simulink model "SMDFR_HTE_model"  (R2024b)
settings: Solver=ode15s  StartTime=1  StopTime=1200  FixedStep=0.01  RelTol=1e-3
model workspace (MAT data in the model file):
  ACS_lambda = 0.000161129786201
  A_cucl = 134.446
  A_cucl2 = 134.446
  A_cuocl = 213.991
  A_d = 217.647058824
  A_fw = [13.6 90 13.6]
  A_h = 217.647058824
  A_h2 = 217.647058824
  A_h20 = 18.015
  A_hcl = 36.458
  A_o = 32
  A_sg = 370
  A_wc = [10.9 103 10.9]
  C_c = 140.2
  C_cucl = 0.71
  C_cuocl = 1
  C_dst = 1996000
  C_h20 = 4.48
  C_hcl = 0.8
  C_hst = 1996000
  C_i0 = [429000000000000; 4.15e+15; 3.83e+15; 1.16e+16; 5.7e+15; 1.53e+15]
  C_o = 0.918
  Ce_i0 = [701000000000000; 5.88e+15; 3.36e+15; 5.09e+15; 820000000000000; 39600000000000]
  Cr = 0.00113148387097
  Cr_m = 8.769
  Cr_m_red = 4.3845
  Cr_red = 0.000565741935484
  D = 0.16
  DPB_lambda = 0.01
  EPB_lambda = 0.01
  E_d = 5
  E_e = 5
  E_h = 5
  E_hte = 5
  G_cucl = 44.778
  G_cucl2 = 44.778
  G_cuocl = 35.6355
  G_h2 = 32
  G_h20 = 10
  G_h20i = 10
  G_h20o = 7
  G_hcl = 12.1426
  G_o = 2.66
  G_s = 27000
  H_valve = 1
  Heat = [18744000 5970000 16956000]
  IPB_lambda = 0.01
  K_d = 500
  K_h = 500
  L = 6
  LOCA1 = 0
  LOCA2 = 0
  LOCA3 = 0
  LOCA4 = 0
  LOCA_p = 0.000161129786201
  LOCA_time = 300
  LOCA_times = [408 453 64 457 317 49 140 274 479 483 79 486 ... (4000 elements, 1000x4)]
  LOPC = 0
  LOPC_p = 0.1
  LOPC_times = [214 478 363 291 271 353 3 392 464 5 413 384 ... (1000 elements, 1000x1)]
  L_ACS = 0.01
  Lambda = 1.05e-06
  M_c = [219.9 7705 219.9]
  M_cucl0 = 44.778
  M_cucl20 = 44.778
  M_f = [307.7 1164 307.7]
  M_h20 = 8
  M_hcl0 = 12.1426
  M_w = [39.3 311 39.3]
  N = 1000
  N_0 = 15000000000000
  Nodes = 3
  P_0 = 100000000
  P_decomposition = 160
  P_hydro = 167
  Pb_acs : object (value not decoded)
  Pb_pipes : object (value not decoded)
  Pi_0 = [0.158 0.6899 0.152]
  Power_lambda = 0.01
  RPB_lambda = 0.01
  T_fw = 300
  T_hpi = 100
  T_st = 900
  Tbar_c0 = 1060
  Tbar_f0 = 1288
  Tc_in = 973
  Tin_c = 973
  Tin_f = 1300
  Tout_c = 1100
  Tout_f = 1300
  V_c = 160
  V_d = 160
  V_dst = 100
  V_h = 160
  V_h2 = 160
  V_hst = 100
  V_s = 100
  V_sg = 100
  age = 0
  ages = [0 50]
  alfa_c = -8.28e-06
  alfa_f = -0.000208
  alpha = 0.9926
  alpha_1 = 1
  alpha_2 = 1
  alpha_3 = 1
  alpha_4 = 1
  beta = 0.00302
  beta_i = [7.91e-05 0.000703 0.000504 0.00117 0.000457 0.00011]
  c_pc = [140.2 140.2 140.2]
  c_pf = [400 400 400]
  c_pw = [690 690 690]
  coolpipes = [2166 2166 0]
  d_c = 10187.40024
  d_dst = 3.14
  d_hst = 3.14
  d_st = 6.123
  demand = [0.661834040547 0.662423385196 0.661244695898 0.663602074493 0.660066006601 0.661244695898 0.662423385196 0.662423385196 0.662423385196 0.661244695898 0.661244695898 0.661244695898 ... (8761 elements, 8761x1)]
  diesel_lambda = 0.01
  eta = 0.4
  fail_threshold = 1244
  file = 'SMDFR_Parameters'
  fuelpipes = 1027
  h_dpo = 6801000
  h_fw = [6546 4305.1 7629.5]
  h_fw_st = 4386450
  h_hpo = 7159680
  h_in = 7000
  h_out = 1000
  h_st_in = 4386450
  h_wc = [27405.4 13833.4 32177.3]
  i = 1
  j = 1
  k_d = 2.7187
  k_e = 2.7187
  k_h = 0.005
  k_hte = 2.7187
  k_sg = 500
  lambda_c = 0.184
  lambda_e = 0.1
  lambda_i = [0.0127 0.03 0.11 0.319 1.18 7.02]
  leakage = 6.5
  mdot_c = [5550.5 5550.5 5550.5]
  mdot_c_value = 5550.5
  mdot_f = [327.7 327.7 327.7]
  mdot_f_value = 327.7
  model = 'SMDFR'
  mu = 50.9722799688
  mu_f = -20.9722799688
  mu_o = 30
  n = 0.45
  nsim = 1
  p_h20 = 40
  phi_tot = 3.61e+21
  rho = 7750
  rho_0 = 0.00111
  rhoex_value = 0
  sigma = 625
  sigma_c = 5
  sigma_f = 5.83095189485
  sigma_o = 3
  step = 0.1
  t = 0.008
  tau_c = 5.43
  tau_e = 10
  tr_fun = cfit
  tr_fun.coeffValues{1}.form = 'pp'
  tr_fun.coeffValues{1}.breaks = [0 34473.8 55158.08 82737.12 122381.99]
  tr_fun.coeffValues{1}.coefs = [2.32060289263e-05  0; 5.70481544439e-06  0.8; 2.97327245618e-06  0.918; 0  1]
  tr_fun.coeffValues{1}.pieces = 4
  tr_fun.coeffValues{1}.order = 2
  tr_fun.coeffValues{1}.dim = 1
  tr_fun.sse = 0
  tr_fun.dfe = 0
  tr_fun.activebounds = 0
  tr_fun.xlim = [0 122381.99]
  tr_fun.fittype.fType = 'linearinterp'
  tr_fun.fittype.fTypename = 'Linear interpolant'
  tr_fun.fittype.fCategory = 'interpolant'
  tr_fun.fittype.defn = 'piecewise polynomial'
  tr_fun.fittype.fFeval = 1
  tr_fun.fittype.args = ['p'; 'x']
  tr_fun.fittype.isEmpty = 0
  tr_fun.fittype.numArgs = 2
  tr_fun.fittype.indep = 'x'
  tr_fun.fittype.depen = 'y'
  tr_fun.fittype.coeff = 'p'
  tr_fun.fittype.fFitoptions = curvefit.linearinterpoptions
  tr_fun.fittype.fFitoptions.ExtrapolationMethod = 'linear'
  tr_fun.fittype.fFitoptions.Method = 'LinearInterpolant'
  tsim = 500
  turbine_fun = cfit
  turbine_fun.coeffValues{1}.form = 'pp'
  turbine_fun.coeffValues{1}.breaks = [0 4067.9084 6687.9172 10273.1924 14892.6816]
  turbine_fun.coeffValues{1}.coefs = [0  0; 1.52671242936e-07  0; 1.17145819099e-06  0.0004; 7.66318492529e-06  0.0046]
  turbine_fun.coeffValues{1}.pieces = 4
  turbine_fun.coeffValues{1}.order = 2
  turbine_fun.coeffValues{1}.dim = 1
  turbine_fun.sse = 0
  turbine_fun.dfe = 0
  turbine_fun.activebounds = 0
  turbine_fun.xlim = [0 14892.6816]
  turbine_fun.fittype.fType = 'linearinterp'
  turbine_fun.fittype.fTypename = 'Linear interpolant'
  turbine_fun.fittype.fCategory = 'interpolant'
  turbine_fun.fittype.defn = 'piecewise polynomial'
  turbine_fun.fittype.fFeval = 1
  turbine_fun.fittype.args = ['p'; 'x']
  turbine_fun.fittype.isEmpty = 0
  turbine_fun.fittype.numArgs = 2
  turbine_fun.fittype.indep = 'x'
  turbine_fun.fittype.depen = 'y'
  turbine_fun.fittype.coeff = 'p'
  turbine_fun.fittype.fFitoptions = curvefit.linearinterpoptions
  turbine_fun.fittype.fFitoptions.ExtrapolationMethod = 'linear'
  turbine_fun.fittype.fFitoptions.Method = 'LinearInterpolant'
  v_rec = 4.16e-09
values from neighbouring files (symbols this model uses):
  ACS1_flow = 25    [Only_Inputs.m]    (also in Simulation_model.m; Simulation_model_complete.m; Simulation_model_hydrogen.m; Simulation_model_hydrogen_parallel.m)
  ACS1_response_time = randi(t_max_r_ACS-t_min_r_ACS)+t_min_r_ACS    [Failure_model.m]    (also in Failure_model_outputs.mat = 36; Only_Inputs.m = ACS1_response_time(indexes))
  ACS2_flow = 25    [Only_Inputs.m]    (also in Simulation_model.m; Simulation_model_complete.m; Simulation_model_hydrogen.m; Simulation_model_hydrogen_parallel.m)
  ACS2_response_time = randi(t_max_r_ACS-t_min_r_ACS)+t_min_r_ACS    [Failure_model.m]    (also in Failure_model_outputs.mat = 49; Only_Inputs.m = ACS2_response_time(indexes); Simulation_model_hydrogen_parallel.m = 0)
  ACS3_flow = 25    [Only_Inputs.m]    (also in Simulation_model.m; Simulation_model_complete.m; Simulation_model_hydrogen.m; Simulation_model_hydrogen_parallel.m)
  ACS3_response_time = randi(t_max_r_ACS-t_min_r_ACS)+t_min_r_ACS    [Failure_model.m]    (also in Failure_model_outputs.mat = 62; Only_Inputs.m = ACS3_response_time(indexes); Simulation_model_hydrogen_parallel.m = 0)
  ACS4_flow = 25    [Only_Inputs.m]    (also in Simulation_model.m; Simulation_model_complete.m; Simulation_model_hydrogen.m; Simulation_model_hydrogen_parallel.m)
  ACS4_response_time = randi(t_max_r_ACS-t_min_r_ACS)+t_min_r_ACS    [Failure_model.m]    (also in Failure_model_outputs.mat = 57; Only_Inputs.m = ACS4_response_time(indexes); Simulation_model_hydrogen_parallel.m = 0)
  ACS_1 = 821    [Failure_model_outputs.mat]    (also in Failure_sim.m = ACS_times(1); Only_Inputs.m = ACS_1(indexes))
  ACS_2 = 1010    [Failure_model_outputs.mat]    (also in Failure_sim.m = ACS_times(2); Only_Inputs.m = ACS_2(indexes); Simulation_model_hydrogen_parallel.m = 1)
  ACS_3 = 926    [Failure_model_outputs.mat]    (also in Failure_sim.m = ACS_times(3); Only_Inputs.m = ACS_3(indexes); Simulation_model_hydrogen_parallel.m = 1)
  ACS_4 = 80    [Failure_model_outputs.mat]    (also in Failure_sim.m = ACS_times(4); Only_Inputs.m = ACS_4(indexes); Simulation_model_hydrogen_parallel.m = 1)
  All_Outputs = 1    [Only_Inputs.m]    (also in Simulation_model.m = 0; Simulation_model_complete.m = 0; Simulation_model_hydrogen.m = 0; Simulation_model_hydrogen_parallel.m = 0)
  EDG1_response_time = randi(t_max_r_EDG-t_min_r_EDG)+t_min_r_EDG    [Failure_model.m]    (also in Failure_model_outputs.mat = 170; Only_Inputs.m = EDG1_response_time(indexes))
  EDG2_response_time = randi(t_max_r_EDG-t_min_r_EDG)+t_min_r_EDG    [Failure_model.m]    (also in Failure_model_outputs.mat = 133; Only_Inputs.m = EDG2_response_time(indexes); Simulation_model_hydrogen_parallel.m = 0)
  EDG_1 = 567    [Failure_model_outputs.mat]    (also in Only_Inputs.m = EDG_1(indexes))
  EDG_2 = 323    [Failure_model_outputs.mat]    (also in Only_Inputs.m = EDG_2(indexes); Simulation_model_hydrogen_parallel.m = 1)
  LHS = 0    [Failure_model_outputs.mat]    (also in Failure_sim.m = 60; Only_Inputs.m = LHS(indexes))
  LOCA1_time = 1200    [Failure_model_outputs.mat]    (also in Failure_sim.m = loca_times(1); Only_Inputs.m = LOCA1_time(indexes))
  LOCA2_time = 1200    [Failure_model_outputs.mat]    (also in Failure_sim.m = loca_times(2); Only_Inputs.m = LOCA2_time(indexes); Simulation_model_hydrogen_parallel.m)
  LOCA3_time = 39    [Failure_model_outputs.mat]    (also in Failure_sim.m = loca_times(3); Only_Inputs.m = LOCA3_time(indexes); Simulation_model_hydrogen_parallel.m = 1200)
  LOCA4_time = 18    [Failure_model_outputs.mat]    (also in Failure_sim.m = loca_times(4); Only_Inputs.m = LOCA4_time(indexes); Simulation_model_hydrogen_parallel.m = 1200)
  MSLB1 = 1200    [Failure_model_outputs.mat]    (also in Failure_sim.m = fix(randsample(x_loca, 1, true, lognorm_pdf)); Only_Inputs.m = MSLB1(indexes))
  MSLB2 = 1200    [Failure_model_outputs.mat]    (also in Failure_sim.m = fix(randsample(x_loca, 1, true, lognorm_pdf)); Only_Inputs.m = MSLB2(indexes); Simulation_model_hydrogen_parallel.m = 0)
  MSLB3 = 1200    [Failure_model_outputs.mat]    (also in Failure_sim.m = fix(randsample(x_loca, 1, true, lognorm_pdf)); Only_Inputs.m = MSLB3(indexes); Simulation_model_hydrogen_parallel.m = 0)
  MSLB4 = 1200    [Failure_model_outputs.mat]    (also in Failure_sim.m = fix(randsample(x_loca, 1, true, lognorm_pdf)); Only_Inputs.m = MSLB4(indexes); Simulation_model_hydrogen_parallel.m = 0)
  PDP11 = 1200    [Failure_model_outputs.mat]    (also in Failure_sim.m = pdp_times(1); Only_Inputs.m = PDP11(indexes))
  PDP11_response_time = randi(t_max_r_EDG-t_min_r_EDG)+t_min_r_EDG    [Failure_model.m]    (also in Failure_model_outputs.mat = 136; Only_Inputs.m = PDP11_response_time(indexes))
  PDP12 = 1200    [Failure_model_outputs.mat]    (also in Failure_sim.m = pdp_times(2); Only_Inputs.m = PDP12(indexes); Simulation_model_hydrogen_parallel.m = 0)
  PDP12_response_time = randi(t_max_r_EDG-t_min_r_EDG)+t_min_r_EDG    [Failure_model.m]    (also in Failure_model_outputs.mat = 119; Only_Inputs.m = PDP12_response_time(indexes); Simulation_model_hydrogen_parallel.m = 0)
  PDP21 = 1200    [Failure_model_outputs.mat]    (also in Failure_sim.m = pdp_times(3); Only_Inputs.m = PDP21(indexes); Simulation_model_hydrogen_parallel.m = 0)
  PDP21_response_time = randi(t_max_r_EDG-t_min_r_EDG)+t_min_r_EDG    [Failure_model.m]    (also in Failure_model_outputs.mat = 17; Only_Inputs.m = PDP21_response_time(indexes); Simulation_model_hydrogen_parallel.m = 0)
  PDP22 = 1200    [Failure_model_outputs.mat]    (also in Failure_sim.m = pdp_times(4); Only_Inputs.m = PDP22(indexes); Simulation_model_hydrogen_parallel.m = 0)
  PDP22_response_time = randi(t_max_r_EDG-t_min_r_EDG)+t_min_r_EDG    [Failure_model.m]    (also in Failure_model_outputs.mat = 120; Only_Inputs.m = PDP22_response_time(indexes); Simulation_model_hydrogen_parallel.m = 0)
  PDP31 = 1200    [Failure_model_outputs.mat]    (also in Failure_sim.m = pdp_times(5); Only_Inputs.m = PDP31(indexes); Simulation_model_hydrogen_parallel.m = 0)
  PDP31_response_time = randi(t_max_r_EDG-t_min_r_EDG)+t_min_r_EDG    [Failure_model.m]    (also in Failure_model_outputs.mat = 65; Only_Inputs.m = PDP31_response_time(indexes); Simulation_model_hydrogen_parallel.m = 0)
  PDP32 = 1200    [Failure_model_outputs.mat]    (also in Failure_sim.m = pdp_times(6); Only_Inputs.m = PDP32(indexes); Simulation_model_hydrogen_parallel.m = 0)
  PDP32_response_time = randi(t_max_r_EDG-t_min_r_EDG)+t_min_r_EDG    [Failure_model.m]    (also in Failure_model_outputs.mat = 28; Only_Inputs.m = PDP32_response_time(indexes); Simulation_model_hydrogen_parallel.m = 0)
  PDP41 = 1200    [Failure_model_outputs.mat]    (also in Failure_sim.m = pdp_times(7); Only_Inputs.m = PDP41(indexes); Simulation_model_hydrogen_parallel.m = 0)
  PDP41_response_time = randi(t_max_r_EDG-t_min_r_EDG)+t_min_r_EDG    [Failure_model.m]    (also in Failure_model_outputs.mat = 24; Only_Inputs.m = PDP41_response_time(indexes); Simulation_model_hydrogen_parallel.m = 0)
  PDP42 = 1200    [Failure_model_outputs.mat]    (also in Failure_sim.m = pdp_times(8); Only_Inputs.m = PDP42(indexes); Simulation_model_hydrogen_parallel.m = 0)
  PDP42_response_time = randi(t_max_r_EDG-t_min_r_EDG)+t_min_r_EDG    [Failure_model.m]    (also in Failure_model_outputs.mat = 164; Only_Inputs.m = PDP42_response_time(indexes); Simulation_model_hydrogen_parallel.m = 0)
  PGA = zeros(N,1)    [Crude_MC.m]    (also in Failure_model_outputs.mat = 0.3; Only_Inputs.m = PGA(indexes); Results.mat = [0.197697697698 0.158618618619 0.354014014014 0.1 0.1 0.4126; Simulation_model_hydrogen_parallel.m = 0)
  Power = 1200    [Failure_model_outputs.mat]    (also in Failure_sim.m = fix(randsample(x_loca, 1, true, lognorm_pdf)); Only_Inputs.m = Power(indexes))
  thermal_failure = 0    [Failure_model_outputs.mat]    (also in Failure_sim.m = 1; Only_Inputs.m = zeros(N,1); Simulation_model_hydrogen_parallel.m)
  thermal_failure_time = 1200    [Failure_model_outputs.mat]    (also in Failure_sim.m = 60; Only_Inputs.m = zeros(N,1); Simulation_model_hydrogen_parallel.m)
libraries: SMDFR_lib x8
(part 1 of 2)
settings Model: Creator=leona  LastModifiedBy=stefanomarchetti
settings OptimizationCC: ReuseModelBlockBuffer=off
settings DebuggingCC: UnconnectedInputMsg=warning  UnconnectedLineMsg=warning
settings ModelReferenceCC: EnableRefExpFcnMdlSchedulingChecks=on
settings RTWCC: GPUComputeCapability=3.5  DLArmComputeVersion=19.05

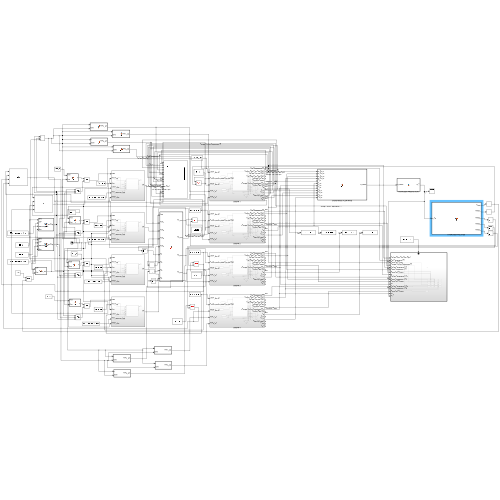
[thumbnail: Simulink's stored preview of the top-level diagram]
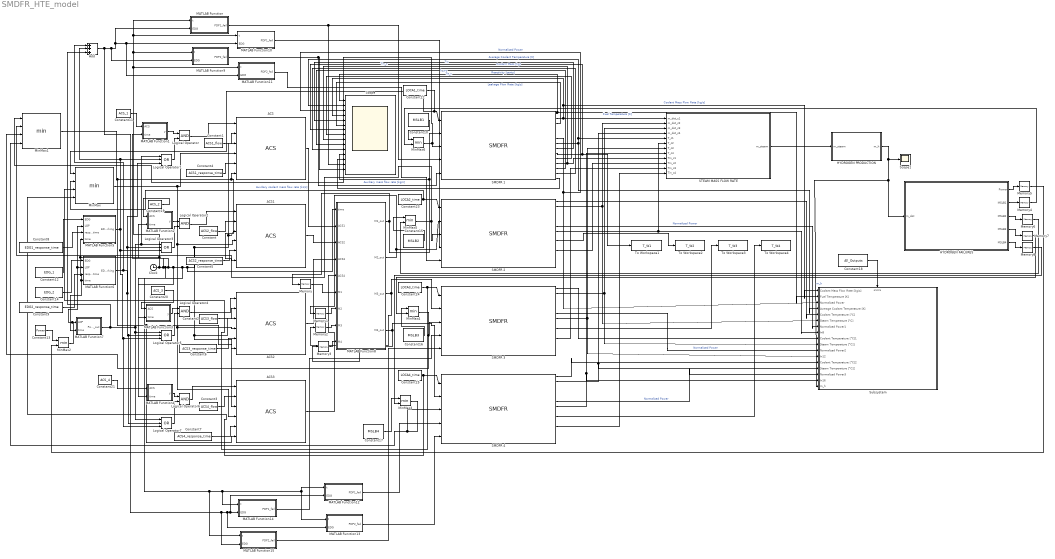
== system SMDFR_HTE_model ==
  ACS{,1..3} (4 alike) : SMDFR_lib/ACS  SystemSampleTime=-1  VariantActivationTime=update diagram  AllowFlexibleInterface=on  Latency=0  AutoFrameSizeCalculation=off
  Add : Sum  Inputs=+++
  Clock : Clock
  Constant : Constant  Value=ACS2_flow
  Constant1 : Constant  Value=ACS1_flow
  Constant10 : Constant  Value=MSLB1
  Constant11 : Constant  Value=ACS_1
  Constant12 : Constant  Value=EDG_1
  Constant13 : Constant  Value=Power
  Constant14 : Constant  Value=EDG_2
  Constant15 : Constant  Value=MSLB2
  Constant16 : Constant  Value=MSLB3
  Constant17 : Constant  Value=MSLB4
  Constant18 : Constant  Value=All_Outputs
  Constant19 : Constant  Value=ACS_2
  Constant2 : Constant  Value=ACS3_flow
  Constant20 : Constant  Value=ACS_3
  Constant21 : Constant  Value=ACS_4
  Constant22 : Constant  Value=LOCA1_time
  Constant23 : Constant  Value=LOCA2_time
  Constant24 : Constant  Value=LOCA3_time
  Constant25 : Constant  Value=LOCA4_time
  Constant3 : Constant  Value=ACS4_flow
  Constant4 : Constant  Value=ACS1_response_time
  Constant5 : Constant  Value=ACS2_response_time
  Constant6 : Constant  Value=ACS3_response_time
  Constant7 : Constant  Value=ACS4_response_time
  Constant8 : Constant  Value=EDG1_response_time
  Constant9 : Constant  Value=EDG2_response_time
  HYDROGEN FAILURES : MATLAB Function  TreatAsAtomicUnit=on
  HYDROGEN PRODUCTION : MATLAB Function  TreatAsAtomicUnit=on
  Logical Operator{,2,4,6} (4 alike) : Logic  AllPortsSameDT=off  OutDataTypeStr=boolean
  Logical Operator{1,3,5,7} (4 alike) : Logic  Operator=OR  Inputs=3  AllPortsSameDT=off  OutDataTypeStr=boolean
  MATLAB Function : MATLAB Function  TreatAsAtomicUnit=on
  MATLAB Function1 : MATLAB Function  TreatAsAtomicUnit=on
  MATLAB Function10 : MATLAB Function  TreatAsAtomicUnit=on
  MATLAB Function11 : MATLAB Function  TreatAsAtomicUnit=on
  MATLAB Function12 : MATLAB Function  TreatAsAtomicUnit=on
  MATLAB Function13 : MATLAB Function  TreatAsAtomicUnit=on
  MATLAB Function14 : MATLAB Function  TreatAsAtomicUnit=on
  MATLAB Function15 : MATLAB Function  TreatAsAtomicUnit=on
  MATLAB Function2 : MATLAB Function  TreatAsAtomicUnit=on
  MATLAB Function3 : MATLAB Function  TreatAsAtomicUnit=on
  MATLAB Function4 : MATLAB Function  TreatAsAtomicUnit=on
  MATLAB Function5 : MATLAB Function  TreatAsAtomicUnit=on
  MATLAB Function6 : MATLAB Function  TreatAsAtomicUnit=on
  MATLAB Function7 : MATLAB Function  TreatAsAtomicUnit=on
  MATLAB Function8 : MATLAB Function  TreatAsAtomicUnit=on
  MATLAB Function9 : MATLAB Function  TreatAsAtomicUnit=on
  Memory{,1..8} (9 alike) : Memory
  MinMax : MinMax  Inputs=4
  MinMax1 : MinMax  Inputs=4
  MinMax{2..6} (5 alike) : MinMax  Inputs=2
  SMDFR 1 : SMDFR_lib/SMDFR  SystemSampleTime=-1  VariantActivationTime=update diagram  AllowFlexibleInterface=on  Latency=0  AutoFrameSizeCalculation=off
  SMDFR 2 : SMDFR_lib/SMDFR  SystemSampleTime=-1  VariantActivationTime=update diagram  AllowFlexibleInterface=on  Latency=0  AutoFrameSizeCalculation=off
      link override SMDFR/SMDFR 1/Constant10: Value=mdot_c_faultcase_2
  SMDFR 3 : SMDFR_lib/SMDFR  SystemSampleTime=-1  VariantActivationTime=update diagram  AllowFlexibleInterface=on  Latency=0  AutoFrameSizeCalculation=off
      link override SMDFR/SMDFR 1/Constant10: Value=mdot_c_faultcase_3
  SMDFR 4 : SMDFR_lib/SMDFR  SystemSampleTime=-1  VariantActivationTime=update diagram  AllowFlexibleInterface=on  Latency=0  AutoFrameSizeCalculation=off
      link override SMDFR/SMDFR 1/Constant10: Value=mdot_c_faultcase_3
  STEAM MASS FLOW RATE : MATLAB Function  TreatAsAtomicUnit=on
  Scope : Scope  NumInputPorts=15
  Scope1 : Scope
  Subsystem : Subsystem
  To Workspace1 : ToWorkspace  VariableName=T_W1  SampleTime=1
  To Workspace2 : ToWorkspace  VariableName=T_W2  SampleTime=1
  To Workspace3 : ToWorkspace  VariableName=T_W3  SampleTime=1
  To Workspace4 : ToWorkspace  VariableName=T_W4  SampleTime=1
  wires:
  SMDFR 1/1 -> Subsystem/2(Fuel Temperature [K]), Scope/1  "Fuel Temperature [K]"
  SMDFR 1/2 -> Subsystem/1(Coolant Mass Flow Rate [kg/s]), Scope/4, STEAM MASS FLOW RATE/1(m_dot_c1)  "Coolant Mass Flow Rate [kg/s]"
  SMDFR 1/6 -> Subsystem/3(Normalized Power), Scope/3  "Normalized Power"
  ACS/1 -> MATLAB Function8/2(ACS1)  "Auxiliary coolant mass flow rate [ks/s]"
  ACS1/1 -> MATLAB Function8/3(ACS2)
  ACS2/1 -> MATLAB Function8/4(ACS3)
  ACS3/1 -> MATLAB Function8/5(ACS4)
  MATLAB Function5/1(EDG_working) -> Logical Operator1/2, Add/2, Logical Operator7/3, Logical Operator5/3, Logical Operator3/3
  Logical Operator1/1 -> Logical Operator/2
  Logical Operator/1 -> ACS/1
  Logical Operator3/1 -> Logical Operator2/2
  MATLAB Function7/1(Power_out) -> Add/3, Logical Operator1/1, Logical Operator3/1, Logical Operator7/1, Logical Operator5/1
  MATLAB Function6/1(EDG_working) -> Add/1, Logical Operator7/2, Logical Operator5/2, Logical Operator1/3, Logical Operator3/2
  Logical Operator2/1 -> ACS1/1
  Logical Operator5/1 -> Logical Operator4/2
  Logical Operator4/1 -> ACS2/1
  Logical Operator7/1 -> Logical Operator6/2
  Logical Operator6/1 -> ACS3/1
  Clock/1 -> MATLAB Function11/1(t), MATLAB Function10/1(t), MATLAB Function/1(t), MATLAB Function9/1(t), MATLAB Function6/4(time), MATLAB Function7/2(time), MATLAB Function5/4(time), MATLAB Function2/2(time), MATLAB Function15/1(t), MATLAB Function14/1(t), MATLAB Function13/1(t), MATLAB Function12/1(t), MATLAB Function1/2(time), MATLAB Function3/2(time), MATLAB Function4/2(time), MATLAB Function8/1(time), ACS1/3, ACS/3, ACS3/3, ACS2/3
  Constant/1 -> ACS1/2
  Constant1/1 -> ACS/2
  Constant2/1 -> ACS2/2
  Constant3/1 -> ACS3/2
  Constant11/1 -> MATLAB Function1/1(ACS)
  Constant19/1 -> MATLAB Function2/1(ACS)
  Constant20/1 -> MATLAB Function3/1(ACS)
  Constant21/1 -> MATLAB Function4/1(ACS)
  Constant22/1 -> MinMax/1, SMDFR 1/1
  Constant23/1 -> SMDFR 2/1, MinMax/2
  Constant24/1 -> MinMax/3, SMDFR 3/1
  Constant25/1 -> SMDFR 4/1, MinMax/4
  MATLAB Function1/1(y) -> Logical Operator/1
  MATLAB Function2/1(y) -> Logical Operator2/1
  MATLAB Function3/1(y) -> Logical Operator4/1
  MATLAB Function4/1(y) -> Logical Operator6/1
  Constant12/1 -> MATLAB Function5/1(EDG)
  Constant14/1 -> MATLAB Function6/1(EDG)
  MinMax2/1 -> MATLAB Function5/2(LOP), MATLAB Function6/2(LOP), MATLAB Function7/1(LOP)
  MATLAB Function8/1(M1_out) -> Memory/1, SMDFR 1/2, Scope/12  "Auxiliary mass flow rate [kg/s]"
  MATLAB Function8/2(M2_out) -> Memory1/1, SMDFR 2/2
  MATLAB Function8/3(M3_out) -> SMDFR 3/2, Memory2/1
  MATLAB Function8/4(M4_out) -> SMDFR 4/2, Memory3/1
  MinMax/1 -> ACS/4, ACS1/4, ACS3/4, ACS2/4
  Constant8/1 -> MATLAB Function5/3(response_time)
  Constant9/1 -> MATLAB Function6/3(response_time)
  Constant4/1 -> ACS/5
  Constant5/1 -> ACS1/5
  Constant6/1 -> ACS2/5
  Constant7/1 -> ACS3/5
  Memory/1 -> MATLAB Function8/6(M1)
  Memory1/1 -> MATLAB Function8/7(M2)
  Memory2/1 -> MATLAB Function8/8(M3)
  Memory3/1 -> MATLAB Function8/9(M4)
  SMDFR 1/7 -> STEAM MASS FLOW RATE/5(T_c1), Scope/2, Subsystem/4(Average Coolant Temperature [K])  "Average Coolant Temperature [K]"
  SMDFR 1/8 -> Scope/5  "Coolant Mass [kg]"
  SMDFR 1/3 -> Scope/6  "Leakage Flow Rate [kg/s]"
  SMDFR 1/9 -> To Workspace1/1, Scope/7  "Tw"
  SMDFR 1/10 -> Scope/8  "Te_c"
  SMDFR 1/11 -> STEAM MASS FLOW RATE/9(Tin_c1), Scope/9  "Tin_c"
  SMDFR 1/12 -> Scope/10  "Reactivity [cents]"
  SMDFR 1/13 -> Scope/11  "h_wc"
  SMDFR 2/9 -> To Workspace2/1
  SMDFR 3/9 -> To Workspace3/1
  SMDFR 4/9 -> To Workspace4/1
  SMDFR 1/14 -> Scope/13
  MATLAB Function/1(PDP1_fail) -> Scope/14, SMDFR 1/4
  MinMax6/1 -> MinMax1/1, SMDFR 1/3
  MinMax5/1 -> SMDFR 2/3, MinMax1/2
  MinMax4/1 -> MinMax1/3, SMDFR 3/3
  MinMax3/1 -> MinMax1/4, SMDFR 4/3
  MATLAB Function10/1(PDP1_fail) -> SMDFR 2/4
  MATLAB Function12/1(PDP1_fail) -> SMDFR 4/4
  MATLAB Function14/1(PDP1_fail) -> SMDFR 3/4
  Add/1 -> MATLAB Function15/2(EDG), MATLAB Function13/2(EDG), MATLAB Function12/2(EDG), MATLAB Function14/2(EDG), MATLAB Function9/2(EDG), MATLAB Function11/2(EDG), MATLAB Function10/2(EDG), MATLAB Function/2(EDG)
  MinMax1/1 -> ACS1/6, ACS/6, ACS2/6, ACS3/6
  MATLAB Function13/1(PDP2_fail) -> SMDFR 4/5
  MATLAB Function15/1(PDP2_fail) -> SMDFR 3/5
  MATLAB Function9/1(PDP2_fail) -> Scope/15, SMDFR 1/5
  MATLAB Function11/1(PDP2_fail) -> SMDFR 2/5
  SMDFR 2/1 -> Subsystem/5(Coolant Temperature [°C])
  SMDFR 2/2 -> STEAM MASS FLOW RATE/2(m_dot_c2), Subsystem/6(Steam Temperature [°C])
  SMDFR 2/6 -> Subsystem/7(Normalized Power1)  "Normalized Power"
  SMDFR 2/7 -> Subsystem/8(In8), STEAM MASS FLOW RATE/6(T_c2)
  SMDFR 3/1 -> Subsystem/9(Coolant Temperature [°C]1)
  SMDFR 3/2 -> STEAM MASS FLOW RATE/3(m_dot_c3), Subsystem/10(Steam Temperature [°C]1)
  SMDFR 3/6 -> Subsystem/11(Normalized Power2)  "Normalized Power"
  SMDFR 3/7 -> STEAM MASS FLOW RATE/7(T_c3), Subsystem/12(In12)
  SMDFR 4/1 -> Subsystem/13(Coolant Temperature [°C]2)
  SMDFR 4/2 -> STEAM MASS FLOW RATE/4(m_dot_c4), Subsystem/14(Steam Temperature [°C]2)
  SMDFR 4/6 -> Subsystem/15(Normalized Power3)  "Normalized Power"
  SMDFR 4/7 -> STEAM MASS FLOW RATE/8(T_c4), Subsystem/16(In16)
  Constant18/1 -> Subsystem/Enable
  STEAM MASS FLOW RATE/1(m_steam) -> HYDROGEN PRODUCTION/1(m_steam)
  HYDROGEN PRODUCTION/1(m_h) -> HYDROGEN FAILURES/1(m_dot), Subsystem/17(m_h), Scope1/1  "m_h"
  SMDFR 2/11 -> STEAM MASS FLOW RATE/10(Tin_c2)
  SMDFR 3/11 -> STEAM MASS FLOW RATE/11(Tin_c3)
  SMDFR 4/11 -> STEAM MASS FLOW RATE/12(Tin_c4)
  Memory5/1 -> MinMax2/2
  Constant13/1 -> MinMax2/1
  Memory8/1 -> MinMax3/2
  Constant17/1 -> MinMax3/1
  Constant16/1 -> MinMax4/1
  Memory7/1 -> MinMax4/2
  Memory6/1 -> MinMax5/2
  Memory4/1 -> MinMax6/2
  Constant10/1 -> MinMax6/1
  Constant15/1 -> MinMax5/1
  HYDROGEN FAILURES/2(MSLB1) -> Memory4/1
  HYDROGEN FAILURES/1(Power) -> Memory5/1
  HYDROGEN FAILURES/3(MSLB2) -> Memory6/1
  HYDROGEN FAILURES/4(MSLB3) -> Memory7/1
  HYDROGEN FAILURES/5(MSLB4) -> Memory8/1
